simulink model "model_evap"  (R2018a)
settings: Solver=VariableStepAuto  StartTime=0.0  StopTime=100  RelTol=1e-3
libraries: simulink x1
settings Model: Creator=Duvan Botello  LastModifiedBy=DANIEL

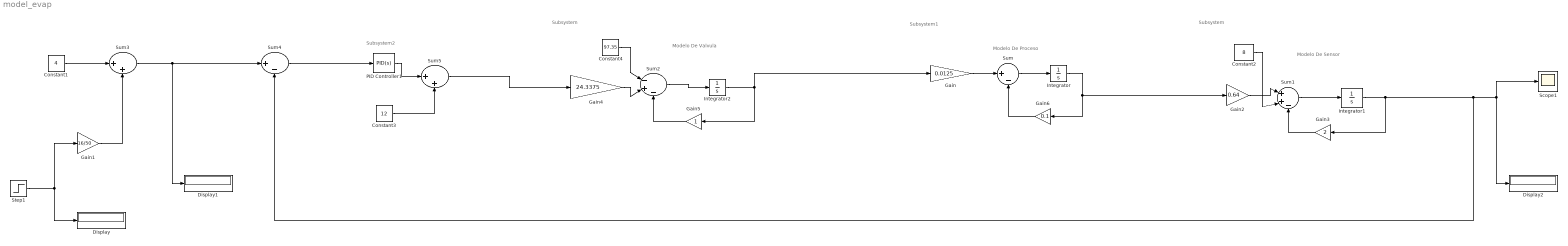
== system model_evap ==
  note: Subsystem2
  note: Subsystem1
  note: Subsystem
  note: Subsystem
  note: Modelo De Sensor
  note: Modelo De Valvula
  note: Modelo De Proceso
  Constant1 : Constant  Value=4
  Constant2 : Constant  Value=8
  Constant3 : Constant  Value=12
  Constant4 : Constant  Value=97.35
  Display : Display
  Display1 : Display
  Display2 : Display
  Gain : Gain  Gain=0.0125
  Gain1 : Gain  Gain=16/50
  Gain2 : Gain  Gain=0.64
  Gain3 : Gain  Gain=2
  Gain4 : Gain  Gain=24.3375
  Gain5 : Gain
  Gain6 : Gain  Gain=0.1
  Integrator : Integrator
  Integrator1 : Integrator
  Integrator2 : Integrator
  PID Controller1 : simulink/Continuous/PID Controller  Controller=PID  TimeDomain=Continuous-time  SampleTime=-1  IntegratorMethod=Forward Euler  FilterMethod=Forward Euler  Form=Parallel  UseFilter=on  ControllerParametersSource=internal  P=7.714  I=0.285  D=0.875  N=100  InitialConditionSource=internal  InitialConditionForIntegrator=0  InitialConditionForFilter=0  ExternalReset=none  LimitOutput=off  UpperSaturationLimit=inf  LowerSaturationLimit=-inf  LinearizeAsGain=on  AntiWindupMode=none  Kb=1  TrackingMode=off  Kt=1  PParamMin=[]  PParamMax=[]  IParamMin=[]  IParamMax=[]  DParamMin=[]  DParamMax=[]  NParamMin=[]  NParamMax=[]  KbParamMin=[]  KbParamMax=[]  KtParamMin=[]  KtParamMax=[]  POutMin=[]  POutMax=[]  IOutMin=[]  IOutMax=[]  DOutMin=[]  DOutMax=[]  NOutMin=[]  NOutMax=[]  KbOutMin=[]  KbOutMax=[]  KtOutMin=[]  KtOutMax=[]  IntegratorOutMin=[]  IntegratorOutMax=[]  FilterOutMin=[]  FilterOutMax=[]  SumOutMin=[]  SumOutMax=[]  SumI1OutMin=[]  SumI1OutMax=[]  SumI2OutMin=[]  SumI2OutMax=[]  SumI3OutMin=[]  SumI3OutMax=[]  SumDOutMin=[]  SumDOutMax=[]  SaturationOutMin=[]  SaturationOutMax=[]  IntegratorContinuousStateAttributes=''  IntegratorStateMustResolveToSignalObject=off  IntegratorRTWStateStorageClass=Auto  FilterContinuousStateAttributes=''  FilterStateMustResolveToSignalObject=off  FilterRTWStateStorageClass=Auto  DifferentiatorICPrevScaledInput=0  DifferentiatorOutMin=[]  DifferentiatorOutMax=[]  FilterDiffOutCoefMin=[]  FilterDiffOutCoefMax=[]  SumDenOutMin=[]  SumDenOutMax=[]  SumNumOutMin=[]  SumNumOutMax=[]  ReciprocalOutMin=[]  ReciprocalOutMax=[]  DivideOutMin=[]  DivideOutMax=[]  TunerSelectOption=Transfer Function Based (PID Tuner App)
  Scope1 : Scope
  Step1 : Step  Time=0  After=10  SampleTime=0
  Sum : Sum  Inputs=|+-
  Sum1 : Sum  Inputs=|++-
  Sum2 : Sum  Inputs=|-+-
  Sum3 : Sum  Inputs=|++
  Sum4 : Sum  Inputs=|+-
  Sum5 : Sum  Inputs=|++
  wires:
  Gain3/1 -> Sum1/3
  Gain2/1 -> Sum1/1
  Constant2/1 -> Sum1/2
  Sum1/1 -> Integrator1/1
  Step1/1 -> Display/1, Gain1/1
  Integrator1/1 -> Gain3/1, Scope1/1, Display2/1, Sum4/2
  Gain1/1 -> Sum3/2
  Constant1/1 -> Sum3/1
  Sum3/1 -> Display1/1, Sum4/1
  Gain4/1 -> Sum2/2
  Sum2/1 -> Integrator2/1
  Constant4/1 -> Sum2/1
  Gain5/1 -> Sum2/3
  Sum/1 -> Integrator/1
  Gain/1 -> Sum/1
  Gain6/1 -> Sum/2
  PID Controller1/1 -> Sum5/1
  Sum4/1 -> PID Controller1/1
  Constant3/1 -> Sum5/2
  Sum5/1 -> Gain4/1
  Integrator2/1 -> Gain5/1, Gain/1
  Integrator/1 -> Gain6/1, Gain2/1
